simulink model "plantaPID"  (R2014a)
settings: Solver=ode45  StartTime=0.0  StopTime=10.0  RelTol=1e-3
libraries: simulink x2
settings Model: Creator=ISRRA  LastModifiedBy=ISRRA

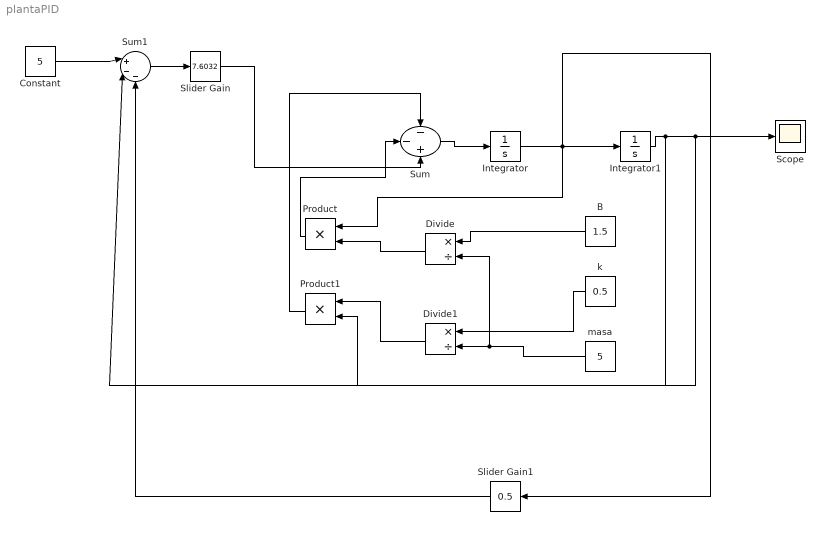
== system plantaPID ==
  "B " : Constant  Value=1.5
  Constant : Constant  Value=5
  Divide : Product  Inputs=*/
  Divide1 : Product  Inputs=*/
  Integrator : Integrator
  Integrator1 : Integrator  InitialCondition=2
  Product : Product
  Product1 : Product
  Scope : Scope
  Slider Gain : simulink/Math Operations/Slider Gain  low=0  gain=7.6032  high=7.6032
  Slider Gain1 : simulink/Math Operations/Slider Gain  low=0  gain=0.5  high=2
  Sum : Sum  Inputs=--+
  Sum1 : Sum  Inputs=|+--
  "k " : Constant  Value=0.5
  "masa " : Constant  Value=5
  wires:
  "B "/1 -> Divide/1
  "k "/1 -> Divide1/1
  "masa "/1 -> Divide/2, Divide1/2
  Divide/1 -> Product/2
  Divide1/1 -> Product1/1
  Product1/1 -> Sum/1
  Product/1 -> Sum/2
  Sum/1 -> Integrator/1
  Constant/1 -> Sum1/1
  Integrator1/1 -> Product1/2, Sum1/2, Scope/1
  Sum1/1 -> Slider Gain/1
  Slider Gain/1 -> Sum/3
  Integrator/1 -> Slider Gain1/1, Product/1, Integrator1/1
  Slider Gain1/1 -> Sum1/3
